simulink model "mpcStep"  (R2023a)
settings: Solver=VariableStepAuto  StartTime=0.0  StopTime=10.0  RelTol=1e-3
values from neighbouring files (symbols this model uses):
  sysdis2 = ssest(pqrDatae,sysdis2,opt)    [greyBox.m]
undefined symbols (not defined in the file or in its folder): sys
libraries: mpclib x1
settings Model: Creator=LENOVO  LastModifiedBy=LENOVO

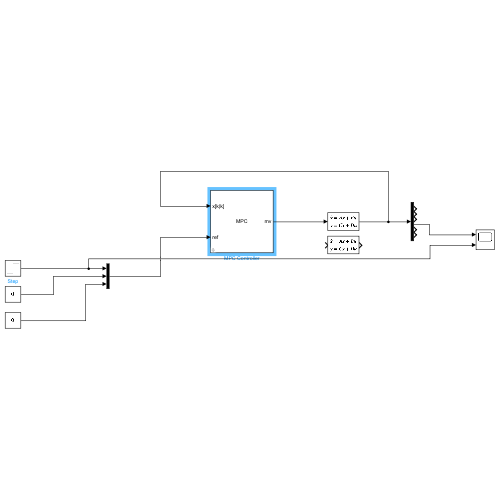
[thumbnail: Simulink's stored preview of the top-level diagram]
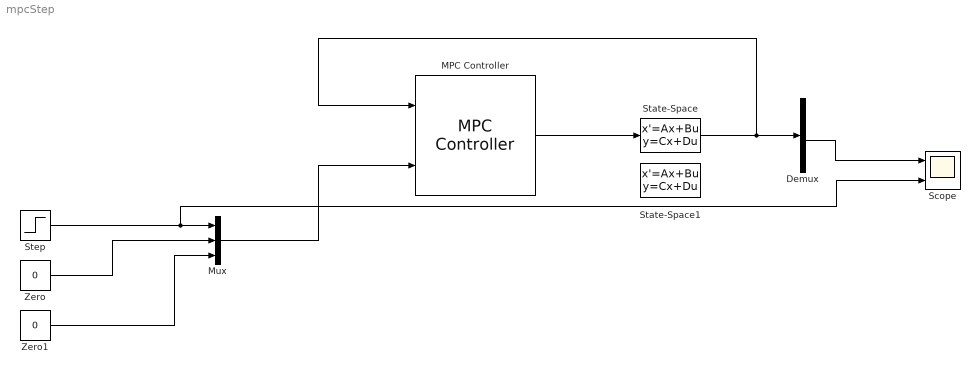
== system mpcStep ==
  Demux : Demux  Outputs=6
  MPC Controller : mpclib/MPC Controller  SCDEnableBlockLinearizationSpecification=on  mpcobj=mpcobj  is_multiple=0  enable_value=0  return_u0=off  updateMPCinCallerWorkspace=on  md_inport=off  mv_inport=off  uref_inport=off  return_cost=off  return_mvseq=off  return_qpstatus=off  return_xseq=off  return_state=off  return_ovseq=off  state_inport=on  umin_inport=off  umax_inport=off  ymin_inport=off  ymax_inport=off  cc_inport=off  ywt_inport=off  uwt_inport=off  duwt_inport=off  rhoeps_inport=off  pm_inport=off  MaximumP=10  HorizonChoice=FixedHorizon  n_ts=0.01  n_p=5  n_mv=3  n_md=0  n_ud=0  n_mo=3  n_uo=0  BlockDataType=double  SampleTimeInherited=off  switch_inport=off
  Mux : Mux  Inputs=3
  Scope : Scope  NumInputPorts=2
  State-Space : StateSpace  A=sysdis2.A  B=sysdis2.B  C=eye(6)  D=zeros(6,3)  InitialCondition=0
  State-Space1 : StateSpace  A=sys.A  B=sys.B  C=eye(6)  D=zeros(6,3)  InitialCondition=0
  Step : Step  SampleTime=0
  Zero : Constant  Value=0  OutDataTypeStr=Inherit: Inherit via back propagation
  Zero1 : Constant  Value=0  OutDataTypeStr=Inherit: Inherit via back propagation
  wires:
  MPC Controller/1 -> State-Space/1
  State-Space/1 -> MPC Controller/1, Demux/1
  Step/1 -> Mux/1, Scope/2
  Zero/1 -> Mux/2
  Zero1/1 -> Mux/3
  Mux/1 -> MPC Controller/2
  Demux/4 -> Scope/1
